simulink model "genSimu"  (R2023a)
settings: Solver=VariableStepAuto  StartTime=0.0  StopTime=inf  RelTol=1e-3
InitFcn:
  | configSimu
StopFcn:
  | disp("End Simulation");
  | COM = get_param("genSimu/generator PID/generator serial configuration", "Port");
  | SP = serialport(COM, 115200);
undefined symbols (not defined in the file): CR, LF
libraries: instrumentseriallib x4, slpidlib x1
settings Model: Creator=zpagg  LastModifiedBy=zpagg

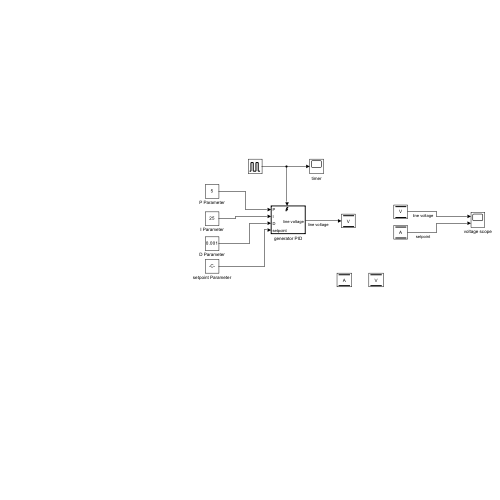
[thumbnail: Simulink's stored preview of the top-level diagram]
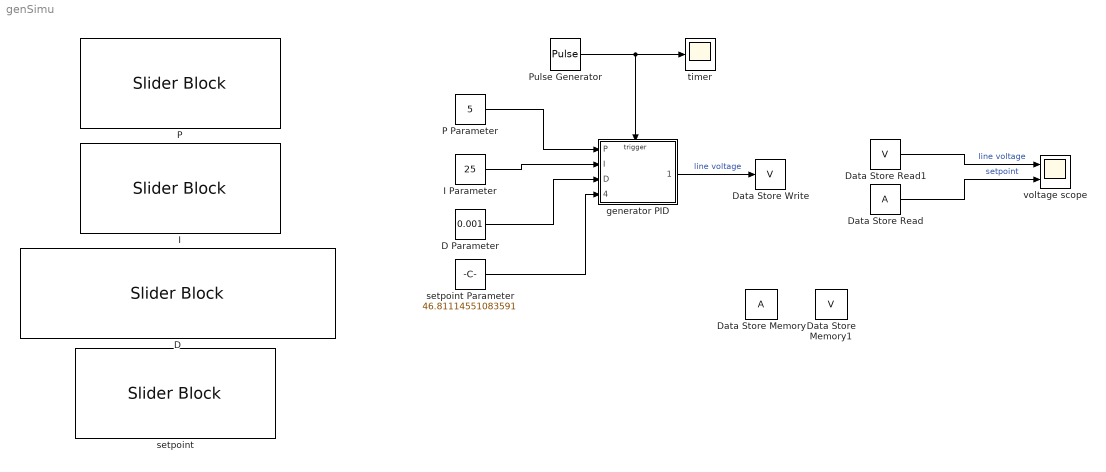
== system genSimu ==
  D : SliderBlock  ScaleMax=5
  D Parameter : Constant  Value=0.001  OutDataTypeStr=single
  Data Store Memory : DataStoreMemory  WriteAfterWriteMsg=warning  ShowAdditionalParam=off
  Data Store Memory1 : DataStoreMemory  DataStoreName=V  WriteAfterWriteMsg=warning  ShowAdditionalParam=off
  Data Store Read : DataStoreRead  IndexOptions=Index vector (dialog)  Indices=1  OutputSizes=1
  Data Store Read1 : DataStoreRead  DataStoreName=V  IndexOptions=Index vector (dialog)  Indices=1  OutputSizes=1
  Data Store Write : DataStoreWrite  DataStoreName=V  IndexOptions=Index vector (dialog)  Indices=1  OutputSizes=1
  I : SliderBlock
  I Parameter : Constant  Value=25  OutDataTypeStr=single
  P : SliderBlock  ScaleMax=50
  P Parameter : Constant  Value=5  OutDataTypeStr=single
  Pulse Generator : DiscretePulseGenerator  PulseType=Time based  Period=0.05  PulseWidth=50  PhaseDelay=1
  generator PID : Subsystem
  setpoint : SliderBlock  ScaleMax=180
  setpoint Parameter : Constant  Value=46.81114551083591
  timer : Scope
  voltage scope : Scope  NumInputPorts=2
  wires:
  Data Store Read/1 -> voltage scope/2  "setpoint"
  P Parameter/1 -> generator PID/1(P)
  I Parameter/1 -> generator PID/2(I)
  D Parameter/1 -> generator PID/3(D)
  Pulse Generator/1 -> timer/1, generator PID/Trigger
  Data Store Read1/1 -> voltage scope/1  "line voltage"
  generator PID/1(line voltage) -> Data Store Write/1  "line voltage"
  setpoint Parameter/1 -> generator PID/4(setpoint)

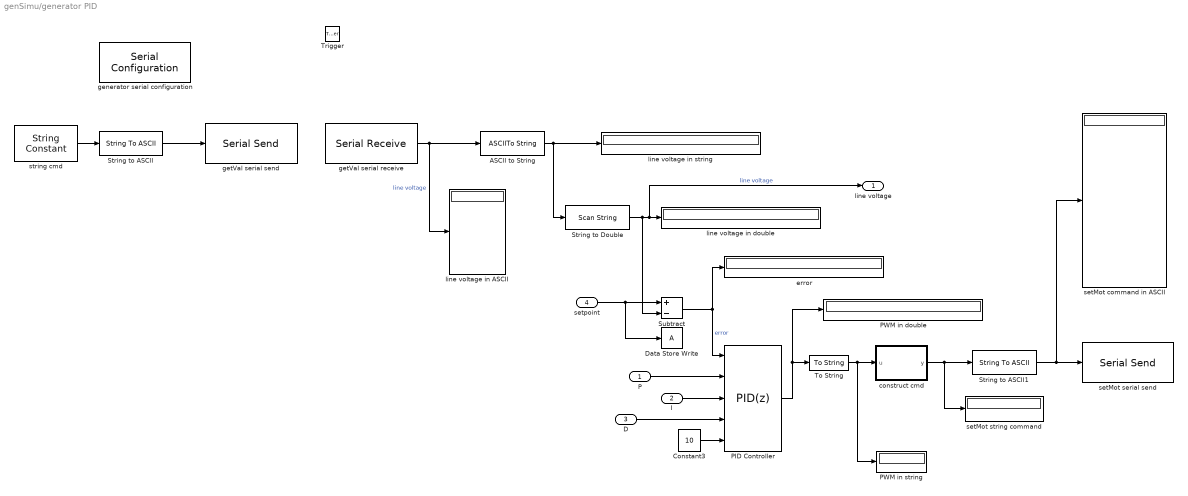
== system genSimu/generator PID ==
  P : Inport
  I : Inport  Port=2
  D : Inport  Port=3
  setpoint : Inport  Port=4
  Trigger : TriggerPort  VariantControl=(inherit)  PortDimensions=1
  ASCII to String : ASCIIToString
  Constant3 : Constant  Value=10  OutDataTypeStr=uint8
  Data Store Write : DataStoreWrite  IndexOptions=Index vector (dialog)  Indices=1  OutputSizes=1
  PID Controller : slpidlib/PID Controller  Controller=PID  Form=Parallel  TimeDomain=Discrete-time  UseExternalTs=off  SampleTime=-1  IntegratorMethod=Forward Euler  FilterMethod=Forward Euler  ControllerParametersSource=external  P=5  I=25  UseKiTs=off  D=0.001  N=10  UseFilter=on  TunerSelectOption=Transfer Function Based (PID Tuner App)  InitialConditionSource=internal  InitialConditionForIntegrator=0  InitialConditionForFilter=0  DifferentiatorICPrevScaledInput=0  ExternalReset=none  TrackingMode=off  Kt=1  LimitOutput=on  SatLimitsSource=internal  UpperSaturationLimit=255  LowerSaturationLimit=0  LinearizeAsGain=off  AntiWindupMode=clamping  Kb=1  LimitIntegrator=on  UpperIntegratorSaturationLimit=255  LowerIntegratorSaturationLimit=0  POutMin=[]  POutMax=[]  IOutMin=[]  IOutMax=[]  DOutMin=[]  DOutMax=[]  NOutMin=[]  NOutMax=[]  SumOutMin=[]  SumOutMax=[]  SaturationOutMin=[]  SaturationOutMax=[]  PParamMin=[]  PParamMax=[]  IParamMin=[]  IParamMax=[]  DParamMin=[]  DParamMax=[]  NParamMin=[]  NParamMax=[]  KbParamMin=[]  KbParamMax=[]  KtParamMin=[]  KtParamMax=[]  KbOutMin=[]  KbOutMax=[]  KtOutMin=[]  KtOutMax=[]  IntegratorOutMin=[]  IntegratorOutMax=[]  FilterOutMin=[]  FilterOutMax=[]  SumI1OutMin=[]  SumI1OutMax=[]  SumI2OutMin=[]  SumI2OutMax=[]  SumI3OutMin=[]  SumI3OutMax=[]  SumI4OutMin=[]  SumI4OutMax=[]  SumDOutMin=[]  SumDOutMax=[]  DifferentiatorOutMin=[]  DifferentiatorOutMax=[]  FilterDiffOutCoefMin=[]  FilterDiffOutCoefMax=[]  ReciprocalOutMin=[]  ReciprocalOutMax=[]  SumDenOutMin=[]  SumDenOutMax=[]  SumNumOutMin=[]  SumNumOutMax=[]  DivideOutMin=[]  DivideOutMax=[]  UdiffTsProdOutMin=[]  UdiffTsProdOutMax=[]  NTsProdOutMin=[]  NTsProdOutMax=[]  UintegralTsProdOutMin=[]  UintegralTsProdOutMax=[]  UngainTsProdOutMin=[]  UngainTsProdOutMax=[]  ClampingZeroOutDataTypeStr=Inherit: Inherit via back propagation  ClampingZeroOutMin=[]  ClampingZeroOutMax=[]  FilterDenConstantOutDataTypeStr=Inherit: Inherit via back propagation  FilterDenConstantOutMin=[]  FilterDenConstantOutMax=[]  PCopyOutDataTypeStr=Inherit: Inherit via back propagation  PCopyOutMin=[]  PCopyOutMax=[]  NCopyOutDataTypeStr=Inherit: Inherit via back propagation  NCopyOutMin=[]  NCopyOutMax=[]  IntegratorContinuousStateAttributes=''  IntegratorStateMustResolveToSignalObject=off  IntegratorRTWStateStorageClass=Auto  FilterContinuousStateAttributes=''  FilterStateMustResolveToSignalObject=off  FilterRTWStateStorageClass=Auto  ParallelPVariant=ExternalParameters  IdealPVariant=Disabled  IVariant=ExternalParameters  DVariant=ExternalParameters  IntegratorVariant=Discrete  SatVariant=Enabled  AWVariant=DiscClampingParallel  PCopyVariant=Disabled  TRVariant=Disabled  FdbkBlocksVariant=Forward  IdealPFdbkVariant=Disabled  SatFdbkVariant=Disabled  DerivativeFilterVariant=ForwardEulerFilter  NVariant=ExternalParameters  NCopyVariant=Disabled  FilterICVariant=InternalICsFilter  IntegratorICVariant=InternalICs  ExternalResetVariant=Disabled  TRSumVariant=Passthrough  SumFdbkVariant=Disabled  SumVariant=Sum_PID  TsampFilterVariant=InternalTs  TsampNgainVariant=Passthrough  TsampIntegralVariant=Disabled_SignalSpec  ExternalSaturationOutDataTypeStr=Inherit: Same as second input
  PWM in double : Display
  PWM in string : Display
  String to ASCII : StringToASCII
  String to ASCII1 : StringToASCII  OutputVectorSize=15
  String to Double : ScanString  Format="\"%lf\""
  Subtract : Sum  Inputs=+-
  To String : ToString
  construct cmd : MATLAB Function  TreatAsAtomicUnit=on
  error : Display
  generator serial configuration : instrumentseriallib/Serial Configuration  Priority=-200000  PortSel=COM23  Port=COM23  ComPort=COM23  BaudRate=115200  DataBits=8  Parity=none  StopBits=1  ByteOrder=little-endian  FlowControl=none  Timeout=2  SimulateUsing=Interpreted execution  BlockInModel=on  aMode=1
  getVal serial receive : instrumentseriallib/Serial Receive  Priority=1  PortSel=COM23  Port=COM23  ComPort=COM23  DataType=uint8  SaveDataType=uint8  ToggleHeader=off  Header=[]  DataSize=[1 6]  ToggleTerminator=on  Terminator=CR/LF ('\r\n')  CustomTerminator=[]  InputFormat=Column major  ToggleDataSize=on  EnableBlockingMode=on  ActionDataUnavailable=Output last received value  ActionWhenDataUnavailable=Output last received value  CustomValue=0  SampleTime=-1  SimulateUsing=Interpreted execution  BlockInModel=on  aMode=1
  getVal serial send : instrumentseriallib/Serial Send  Priority=1  PortSel=COM23  Port=COM23  ComPort=COM23  Header=[]  Terminator=LF ('\n')  CustomTerminator=[]  EnableBlockingMode=on  SimulateUsing=Interpreted execution  BlockInModel=on  aMode=1
  line voltage in ASCII : Display
  line voltage in double : Display
  line voltage in string : Display
  setMot command in ASCII : Display
  setMot serial send : instrumentseriallib/Serial Send  Priority=1  PortSel=COM23  Port=COM23  ComPort=COM23  Header=[]  Terminator=LF ('\n')  CustomTerminator=[]  EnableBlockingMode=on  SimulateUsing=Interpreted execution  BlockInModel=on  aMode=1
  setMot string command : Display
  string cmd : StringConstant  String="\"getVal\""
  line voltage : Outport
  wires:
  String to ASCII/1 -> getVal serial send/1
  string cmd/1 -> String to ASCII/1
  getVal serial receive/1 -> line voltage in ASCII/1, ASCII to String/1  "line voltage"
  ASCII to String/1 -> String to Double/1, line voltage in string/1
  String to Double/1 -> Subtract/2, line voltage/1, line voltage in double/1  "line voltage"
  Subtract/1 -> error/1, PID Controller/1  "error"
  PID Controller/1 -> PWM in double/1, To String/1
  To String/1 -> PWM in string/1, construct cmd/1(u)
  construct cmd/1(y) -> String to ASCII1/1, setMot string command/1
  String to ASCII1/1 -> setMot command in ASCII/1, setMot serial send/1
  P/1 -> PID Controller/2
  Constant3/1 -> PID Controller/5
  setpoint/1 -> Data Store Write/1, Subtract/1
  I/1 -> PID Controller/3
  D/1 -> PID Controller/4

== matlab function genSimu/generator PID/construct cmd ==
  data: u input; y output
function y = fcn(u)
y = "setMot" + newline + u;
